simulink model "BicyclePeterCorkeP2P"  (R2021a)
settings: Solver=VariableStepAuto  StartTime=0.0  StopTime=30  RelTol=1e-3
values from neighbouring files (symbols this model uses):
  accelLim = 1    [BicyclePeterCorkeP2PSetup.m]
  goalCoord = [5 5]    [BicyclePeterCorkeP2PSetup.m]
  initCoord = [8 5 2*pi/3]    [BicyclePeterCorkeP2PSetup.m]
  speedLim = 1    [BicyclePeterCorkeP2PSetup.m]
  steerLim = 1    [BicyclePeterCorkeP2PSetup.m]
  wheelBase = 1    [BicyclePeterCorkeP2PSetup.m]
libraries: simulink x2
settings Model: Creator=guyot  LastModifiedBy=User

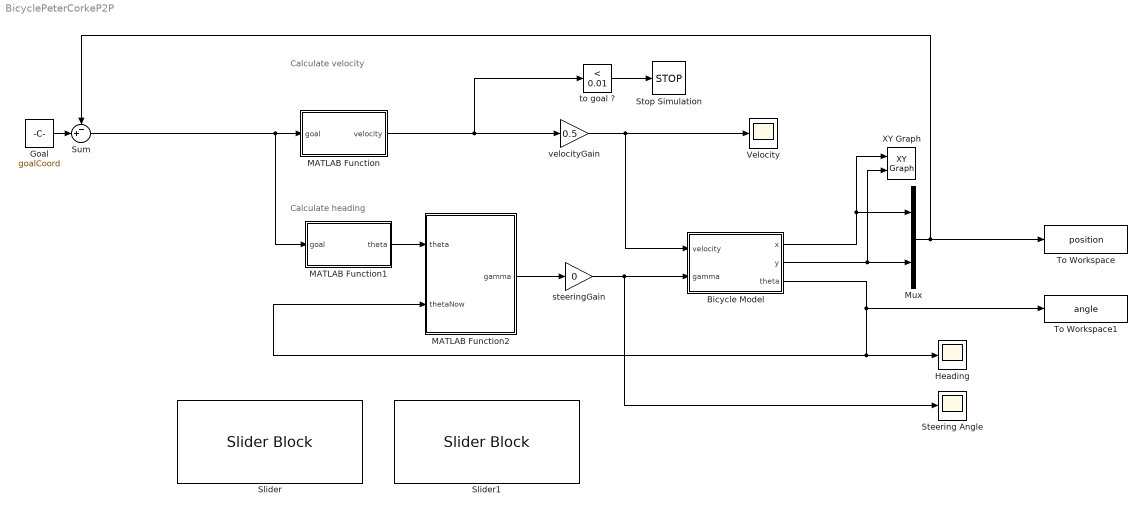
== system BicyclePeterCorkeP2P ==
  note: Calculate heading
  note: Calculate velocity
  Bicycle Model : Subsystem
  Goal : Constant  Value=goalCoord
  Heading : Scope
  MATLAB Function : MATLAB Function  TreatAsAtomicUnit=on
  MATLAB Function1 : MATLAB Function  TreatAsAtomicUnit=on
  MATLAB Function2 : MATLAB Function  TreatAsAtomicUnit=on
  Mux : Mux  Inputs=2
  Slider : SliderBlock  ScaleMax=2
  Slider1 : SliderBlock  ScaleMax=5
  Steering Angle : Scope
  Stop Simulation : Stop
  Sum : Sum  Inputs=-+|
  To Workspace : ToWorkspace  VariableName=position  SaveFormat=Timeseries  SampleTime=-1
  To Workspace1 : ToWorkspace  VariableName=angle  SaveFormat=Timeseries  SampleTime=-1
  Velocity : Scope
  XY Graph : simulink/Sinks/XY Graph  xmin=-2  xmax=10  ymin=-2  ymax=10  st=-1
  steeringGain : Gain  Gain=0
  to goal ? : simulink/Logic and Bit Operations/Compare To Constant  relop=<  const=0.01  OutDataTypeStr=boolean
  velocityGain : Gain  Gain=0.5
  wires:
  Goal/1 -> Sum/2
  MATLAB Function/1(velocity) -> to goal ?/1, velocityGain/1
  velocityGain/1 -> Bicycle Model/1(velocity), Velocity/1
  MATLAB Function1/1(theta) -> MATLAB Function2/1(theta)
  MATLAB Function2/1(gamma) -> steeringGain/1
  steeringGain/1 -> Steering Angle/1, Bicycle Model/2(gamma)
  to goal ?/1 -> Stop Simulation/1
  Bicycle Model/1(x) -> Mux/1, XY Graph/1
  Bicycle Model/2(y) -> XY Graph/2, Mux/2
  Sum/1 -> MATLAB Function1/1(goal), MATLAB Function/1(goal)
  Bicycle Model/3(theta) -> To Workspace1/1, MATLAB Function2/2(thetaNow), Heading/1
  Mux/1 -> To Workspace/1, Sum/1

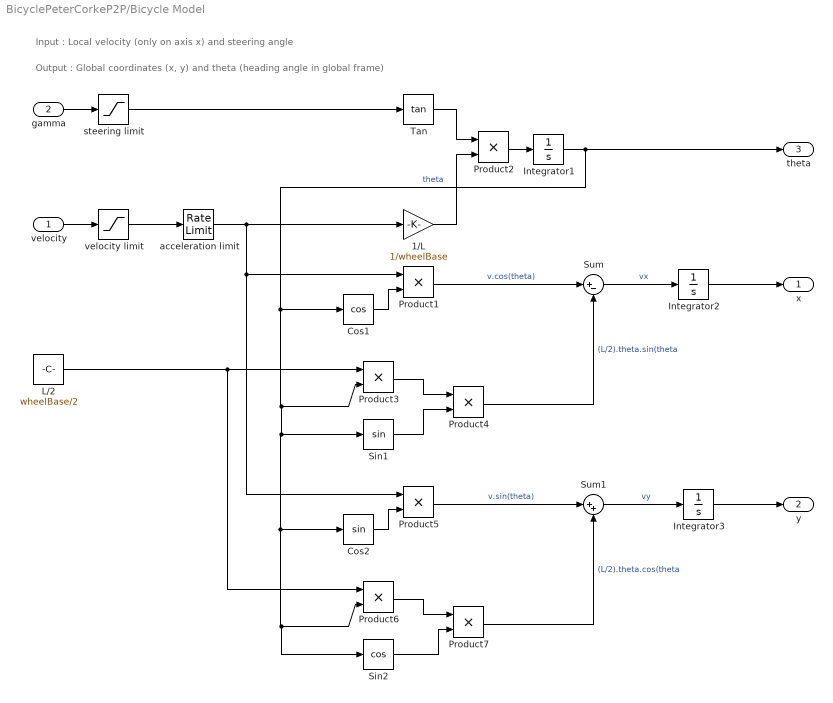
== system BicyclePeterCorkeP2P/Bicycle Model ==
  note: Output : Global coordinates (x, y) and theta (heading angle in global frame)
  note: Input : Local velocity (only on axis x) and steering angle
  velocity : Inport
  gamma : Inport  Port=2
  1/L : Gain  Gain=1/wheelBase
  Cos1 : Trigonometry  Operator=cos
  Cos2 : Trigonometry
  Integrator1 : Integrator  InitialCondition=initCoord(3)
  Integrator2 : Integrator  InitialCondition=initCoord(1)
  Integrator3 : Integrator  InitialCondition=initCoord(2)
  L/2 : Constant  Value=wheelBase/2
  Product{1..7} (7 alike) : Product
  Sin1 : Trigonometry
  Sin2 : Trigonometry  Operator=cos
  Sum : Sum  Inputs=|+-
  Sum1 : Sum  Inputs=|++
  Tan : Trigonometry  Operator=tan
  acceleration limit : RateLimiter  RisingSlewLimit=accelLim  FallingSlewLimit=-accelLim  SampleTimeMode=inherited
  steering limit : Saturate  UpperLimit=steerLim  LowerLimit=-steerLim  ZeroCross=off
  velocity limit : Saturate  UpperLimit=speedLim  LowerLimit=-speedLim
  x : Outport
  y : Outport  Port=2
  theta : Outport  Port=3
  wires:
  velocity limit/1 -> acceleration limit/1
  gamma/1 -> steering limit/1
  steering limit/1 -> Tan/1
  acceleration limit/1 -> Product5/1, Product1/1, 1/L/1
  Cos1/1 -> Product1/2
  Product2/1 -> Integrator1/1
  Product1/1 -> Sum/1  "v.cos(theta)"
  Product3/1 -> Product4/1
  Sin1/1 -> Product4/2
  Product4/1 -> Sum/2  "(L/2).theta.sin(theta"
  Sum/1 -> Integrator2/1  "vx"
  L/2/1 -> Product6/1, Product3/1
  Integrator1/1 -> Cos1/1, Cos2/1, Sin2/1, Product6/2, Sin1/1, Product3/2, theta/1  "theta"
  velocity/1 -> velocity limit/1
  Product7/1 -> Sum1/2  "(L/2).theta.cos(theta"
  Sum1/1 -> Integrator3/1  "vy"
  Sin2/1 -> Product7/2
  Cos2/1 -> Product5/2
  Product5/1 -> Sum1/1  "v.sin(theta)"
  Product6/1 -> Product7/1
  Integrator2/1 -> x/1
  Integrator3/1 -> y/1
  1/L/1 -> Product2/2
  Tan/1 -> Product2/1

== matlab function BicyclePeterCorkeP2P/MATLAB Function ==
  data: goal input; velocity output
function velocity = speedGoal(goal)

velocity = sqrt(goal(1)^2+goal(2)^2);

== matlab function BicyclePeterCorkeP2P/MATLAB Function2 ==
  data: theta input; gamma output; thetaNow input
function gamma = gammaGoal(theta, thetaNow)

gamma = angdiff(thetaNow, theta);

== matlab function BicyclePeterCorkeP2P/MATLAB Function1 ==
  data: goal input; theta output
function theta = goalAngle(goal)

theta = atan2(goal(2),goal(1));
